simulink model "ThrottlePositionControlComposition_TestHarness"  (R2025a)
settings: Solver=FixedStepDiscrete  StartTime=0.0  StopTime=10.0  RelTol=1e-3  EnableMultiTasking=on
settings Model: Creator=z004f2se  LastModifiedBy=z004f2se
settings SolverCC: AutoInsertRateTranBlk=on
settings DataIOCC: SaveFormat=StructureWithTime
settings OptimizationCC: DefaultParameterBehavior=Inlined  EnhancedBackFolding=on  PassReuseOutputArgsAs=Individual arguments  ZeroExternalMemoryAtStartup=off  ZeroInternalMemoryAtStartup=off  OptimizeBlockOrder=speed  DifferentSizesBufferReuse=on  OptimizationCustomize=off  EfficientTunableParamExpr=on
settings DebuggingCC: ParameterTunabilityLossMsg=error
settings ModelReferenceCC: ModelReferenceNumInstancesAllowed=Single
settings SFSimCC: SimGenImportedTypeDefs=on  MATLABDynamicMemAlloc=off
settings RTWCC: SystemTargetFile=autosar.tlc  GenCodeOnly=on  TemplateMakefile=ert_default_tmf  DataTypeReplacement=CDataTypesFixedWidth  Description=AUTOSAR
settings CodeAppCC: ForceParamTrailComments=on  IgnoreCustomStorageClasses=off  OperatorAnnotations=on  SimulinkDataObjDesc=on  SFDataObjDesc=on  InsertBlockDesc=on
settings STFCustomTargetCC: SystemTargetFile=autosar.tlc  TargetLangStandard=C99 (ISO)  MultiwordLength=256.0  DynamicStringBufferSize=256.0  ParMdlRefBuildCompliant=on  CompOptLevelCompliant=on  IncludeMdlTerminateFcn=off  CombineOutputUpdateFcns=on  SuppressErrorStatus=on  ERTCustomFileBanners=on  SubcomponentCodeInterfacePackaging=Nonreusable function  SupportNonFinite=off  SupportComplex=off  SupportContinuousTime=off  SupportNonInlinedSFcns=off  RemoveResetFunc=on  MATLABClassNameForMDSCustomization=Simulink.SoftwareTarget.ERTCustomization  AutosarCompliant=on  GRTInterface=off  UseToolchainInfoCompliant=on  LookupTableObjectStructAxisOrder=2,1,3,4,...  LUTObjectStructOrderEvenSpacing=Size,Table,Breakpoints  AutosarCompilerAbstraction=off  AutosarMatrixIOAsArray=off  AutosarSchemaVersion=4.2  DisableAUTOSARRoutinesHostLibrary=off  AutosarMaxShortNameLength=128.0
settings ERTTargetCC: ExtModeTransport=0.0  ExtModeStaticAlloc=off  ExtModeMexFile=ext_comm  ExtModeIntrfLevel=Level1  ERTCustomFileTemplate=example_file_process.tlc  BooleanTrueId=TRUE  BooleanFalseId=FALSE  TargetLangStandard=C99 (ISO)  ConcurrentExecutionCompliant=off  IncludeMdlTerminateFcn=off  SuppressErrorStatus=on  SubcomponentCodeInterfacePackaging=Nonreusable function  SupportNonFinite=off  SupportComplex=off  ModelStepFunctionPrototypeControlCompliant=off  CPPClassGenCompliant=off  AutosarCompliant=on  LookupTableObjectStructAxisOrder=2,1,3,4,...  LUTObjectStructOrderEvenSpacing=Size,Table,Breakpoints

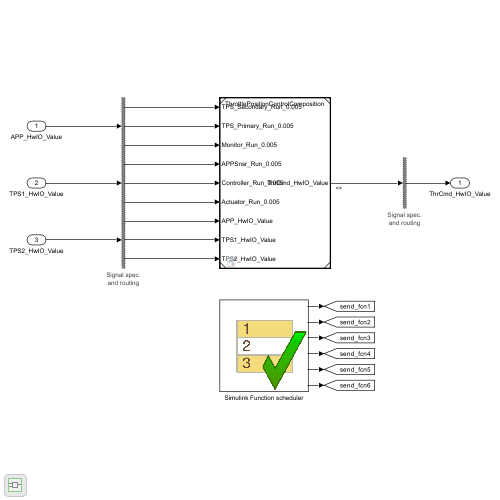
[thumbnail: Simulink's stored preview of the top-level diagram]
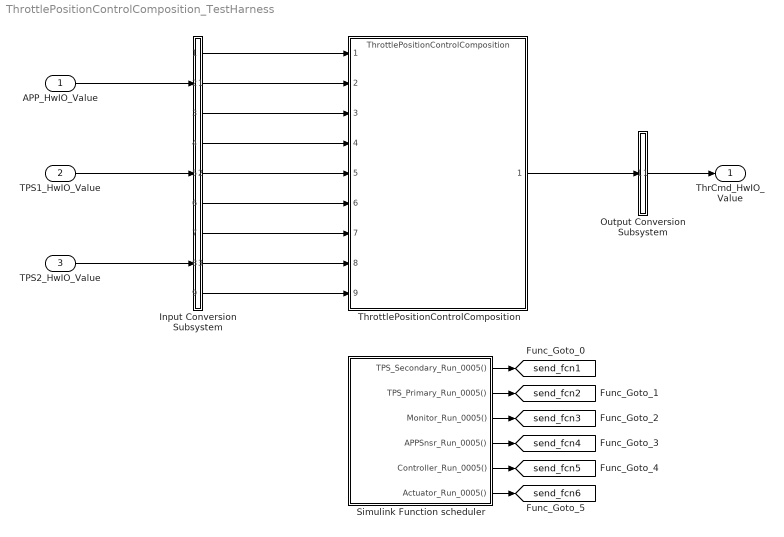
== system ThrottlePositionControlComposition_TestHarness ==
  APP_HwIO_Value : Inport  OutDataTypeStr=uint16  PortDimensions=[1]
  TPS1_HwIO_Value : Inport  Port=2  OutDataTypeStr=uint16  PortDimensions=[1]
  TPS2_HwIO_Value : Inport  Port=3  OutDataTypeStr=uint16  PortDimensions=[1]
  Input Conversion Subsystem : Subsystem  Tag=__SLT_ICS__  Description=|
      | Signal spec.
      | and routing
      settings: AttributesFormatString=%<Description>
  Output Conversion Subsystem : Subsystem  Tag=__SLT_OCS__  Description=|
      | Signal spec.
      | and routing
      settings: AttributesFormatString=%<Description>
  Simulink Function scheduler : Test Sequence  Tag=__SLT_FCN_CALL__  TreatAsAtomicUnit=on
  ThrottlePositionControlComposition : ModelReference  ModelNameDialog=ThrottlePositionControlComposition  SimulationMode=Normal  ScheduleRates=on  ModelReferenceVersion=1.1
  ThrCmd_HwIO_Value : Outport
  tag scope: send_fcn1=global, send_fcn2=global, send_fcn3=global, send_fcn4=global, send_fcn5=global, send_fcn6=global
  wires:
  APP_HwIO_Value/1 -> Input Conversion Subsystem/1(Inport_1)
  TPS1_HwIO_Value/1 -> Input Conversion Subsystem/2(Inport_2)
  TPS2_HwIO_Value/1 -> Input Conversion Subsystem/3(Inport_3)
  Output Conversion Subsystem/1(Outport_1) -> ThrCmd_HwIO_Value/1
  Input Conversion Subsystem/1(Outport_1) -> ThrottlePositionControlComposition/1
  Input Conversion Subsystem/2(Outport_2) -> ThrottlePositionControlComposition/2
  Input Conversion Subsystem/3(Outport_3) -> ThrottlePositionControlComposition/3
  Input Conversion Subsystem/4(Outport_4) -> ThrottlePositionControlComposition/4
  Input Conversion Subsystem/5(Outport_5) -> ThrottlePositionControlComposition/5
  Input Conversion Subsystem/6(Outport_6) -> ThrottlePositionControlComposition/6
  Input Conversion Subsystem/7(Outport_7) -> ThrottlePositionControlComposition/7
  Input Conversion Subsystem/8(Outport_8) -> ThrottlePositionControlComposition/8
  Input Conversion Subsystem/9(Outport_9) -> ThrottlePositionControlComposition/9
  ThrottlePositionControlComposition/1 -> Output Conversion Subsystem/1(Inport_1)
  Simulink Function scheduler/1(TPS_Secondary_Run_0005()) -> [send_fcn1]
  Simulink Function scheduler/2(TPS_Primary_Run_0005()) -> [send_fcn2]
  Simulink Function scheduler/3(Monitor_Run_0005()) -> [send_fcn3]
  Simulink Function scheduler/4(APPSnsr_Run_0005()) -> [send_fcn4]
  Simulink Function scheduler/5(Controller_Run_0005()) -> [send_fcn5]
  Simulink Function scheduler/6(Actuator_Run_0005()) -> [send_fcn6]

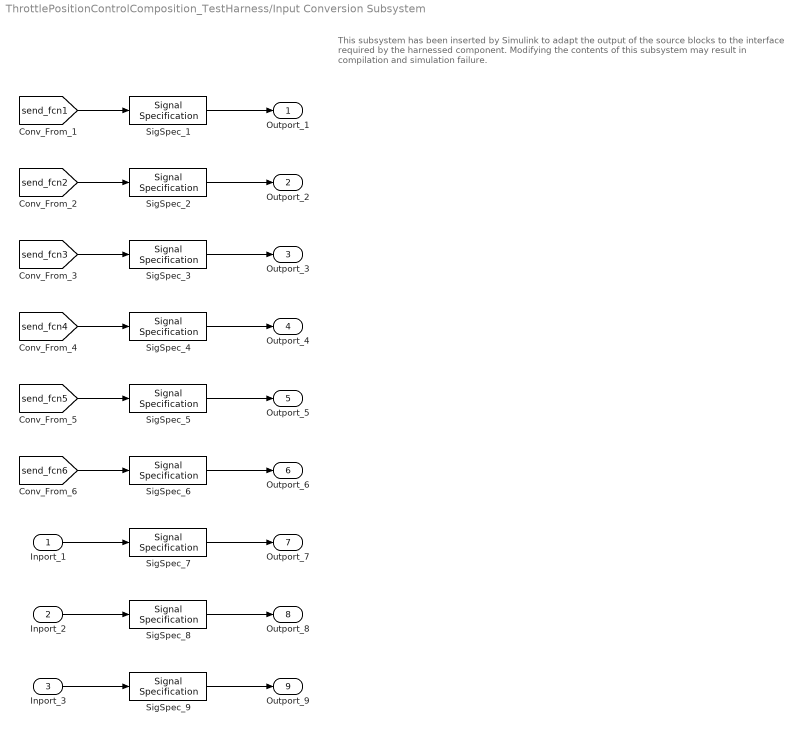
== system ThrottlePositionControlComposition_TestHarness/Input Conversion Subsystem ==
  note: This subsystem has been inserted by Simulink to adapt the output of the source blocks to the interface required by the harnessed component.
      |  Modifying the contents of this subsystem may result in compilation and simulation failure.
  Inport_1 : Inport
  Inport_2 : Inport  Port=2
  Inport_3 : Inport  Port=3
  SigSpec_{1..6} (6 alike) : SignalSpecification
  SigSpec_7 : SignalSpecification  OutDataTypeStr=uint16  Dimensions=[1]
  SigSpec_8 : SignalSpecification  OutDataTypeStr=uint16  Dimensions=[1]
  SigSpec_9 : SignalSpecification  OutDataTypeStr=uint16  Dimensions=[1]
  Outport_1 : Outport
  Outport_2 : Outport  Port=2
  Outport_3 : Outport  Port=3
  Outport_4 : Outport  Port=4
  Outport_5 : Outport  Port=5
  Outport_6 : Outport  Port=6
  Outport_7 : Outport  Port=7
  Outport_8 : Outport  Port=8
  Outport_9 : Outport  Port=9
  wires:
  SigSpec_1/1 -> Outport_1/1
  [send_fcn1] -> SigSpec_1/1
  SigSpec_2/1 -> Outport_2/1
  [send_fcn2] -> SigSpec_2/1
  SigSpec_3/1 -> Outport_3/1
  [send_fcn3] -> SigSpec_3/1
  SigSpec_4/1 -> Outport_4/1
  [send_fcn4] -> SigSpec_4/1
  SigSpec_5/1 -> Outport_5/1
  [send_fcn5] -> SigSpec_5/1
  SigSpec_6/1 -> Outport_6/1
  [send_fcn6] -> SigSpec_6/1
  SigSpec_7/1 -> Outport_7/1
  Inport_1/1 -> SigSpec_7/1
  SigSpec_8/1 -> Outport_8/1
  Inport_2/1 -> SigSpec_8/1
  SigSpec_9/1 -> Outport_9/1
  Inport_3/1 -> SigSpec_9/1

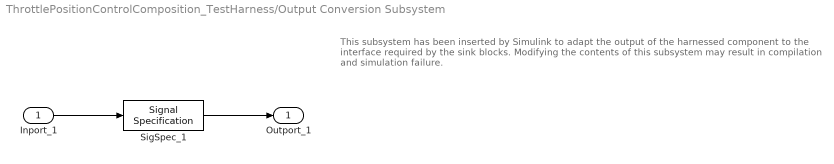
== system ThrottlePositionControlComposition_TestHarness/Output Conversion Subsystem ==
  note: This subsystem has been inserted by Simulink to adapt the output of the harnessed component to the interface required by the sink blocks.
      |  Modifying the contents of this subsystem may result in compilation and simulation failure.
  Inport_1 : Inport
  SigSpec_1 : SignalSpecification  OutDataTypeStr=int16  Dimensions=[1]
  Outport_1 : Outport
  wires:
  Inport_1/1 -> SigSpec_1/1
  SigSpec_1/1 -> Outport_1/1

== stateflow chart ThrottlePositionControlComposition_TestHarness/Simulink Function scheduler ==
  settings: updateMethod=DISCRETE  sampleTime=0.005
  state Run
    send(TPS_Secondary_Run_0005);
    send(TPS_Primary_Run_0005);
    send(Monitor_Run_0005);
    send(APPSnsr_Run_0005);
    send(Controller_Run_0005);
    send(Actuator_Run_0005);
  (default) -> Run
  events: TPS_Secondary_Run_0005 output FUNCTION_CALL_EVENT; TPS_Primary_Run_0005 output FUNCTION_CALL_EVENT; Monitor_Run_0005 output FUNCTION_CALL_EVENT; APPSnsr_Run_0005 output FUNCTION_CALL_EVENT; Controller_Run_0005 output FUNCTION_CALL_EVENT; Actuator_Run_0005 output FUNCTION_CALL_EVENT
